simulink model "Tanque01"  (R2024a)
settings: Solver=VariableStepAuto  StartTime=0.0  StopTime=3600*tf  RelTol=1e-3
undefined symbols (not defined in the file): Dsm, DT, h0
settings Model: Creator=Rodolfo  LastModifiedBy=Rodolfo

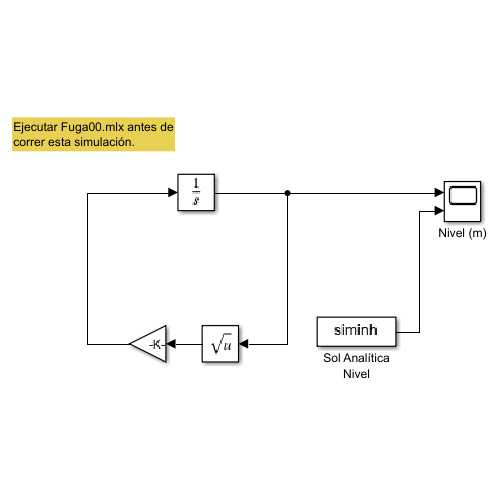
[thumbnail: Simulink's stored preview of the top-level diagram]
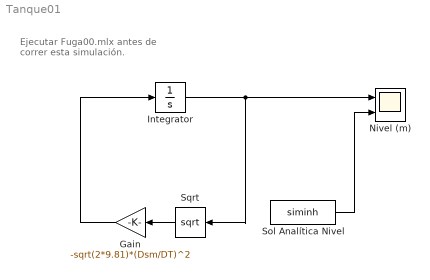
== system Tanque01 ==
  note: Ejecutar Fuga00.mlx antes de
      | correr esta simulación.
  Gain : Gain  Gain=-sqrt(2*9.81)*(Dsm/DT)^2
  Integrator : Integrator  InitialCondition=h0
  Nivel (m) : Scope  NumInputPorts=2
  Sol Analítica Nivel : FromWorkspace  VariableName=siminh
  Sqrt : Sqrt
  wires:
  Integrator/1 -> Sqrt/1, Nivel (m)/1
  Sol Analítica Nivel/1 -> Nivel (m)/2
  Sqrt/1 -> Gain/1
  Gain/1 -> Integrator/1
